simulink model "Fullorder_with_PID"  (R2015b)
settings: Solver=VariableStepAuto  StartTime=0.0  StopTime=10.0  RelTol=1e-3
undefined symbols (not defined in the file): J_pro, Kt, Kv, L, R
libraries: simulink x1
settings Model: Creator=Morten  LastModifiedBy=Morten

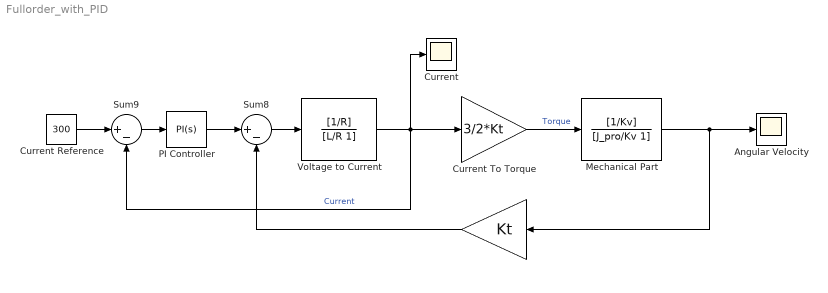
== system Fullorder_with_PID ==
  "                " : Gain  Gain=Kt
  Angular Velocity : Scope
  Current : Scope
  Current Reference : Constant  Value=300
  "Current To Torque " : Gain  Gain=3/2*Kt
  "Mechanical Part " : TransferFcn  Numerator=[1/Kv]  Denominator=[J_pro/Kv 1]
  "PI Controller " : simulink/Continuous/PID Controller  Controller=PI  TimeDomain=Continuous-time  SampleTime=-1  IntegratorMethod=Forward Euler  FilterMethod=Forward Euler  Form=Parallel  UseFilter=on  ControllerParametersSource=internal  P=0.0157  I=2.5637  D=0  N=100  InitialConditionSource=internal  InitialConditionForIntegrator=0  InitialConditionForFilter=0  ExternalReset=none  LimitOutput=off  UpperSaturationLimit=inf  LowerSaturationLimit=-inf  LinearizeAsGain=on  AntiWindupMode=none  Kb=1  TrackingMode=off  Kt=1  PParamMin=[]  PParamMax=[]  IParamMin=[]  IParamMax=[]  DParamMin=[]  DParamMax=[]  NParamMin=[]  NParamMax=[]  KbParamMin=[]  KbParamMax=[]  KtParamMin=[]  KtParamMax=[]  POutMin=[]  POutMax=[]  IOutMin=[]  IOutMax=[]  DOutMin=[]  DOutMax=[]  NOutMin=[]  NOutMax=[]  KbOutMin=[]  KbOutMax=[]  KtOutMin=[]  KtOutMax=[]  IntegratorOutMin=[]  IntegratorOutMax=[]  FilterOutMin=[]  FilterOutMax=[]  SumOutMin=[]  SumOutMax=[]  SumI1OutMin=[]  SumI1OutMax=[]  SumI2OutMin=[]  SumI2OutMax=[]  SumI3OutMin=[]  SumI3OutMax=[]  SumDOutMin=[]  SumDOutMax=[]  SaturationOutMin=[]  SaturationOutMax=[]  IntegratorContinuousStateAttributes=''  IntegratorStateMustResolveToSignalObject=off  IntegratorRTWStateStorageClass=Auto  FilterContinuousStateAttributes=''  FilterStateMustResolveToSignalObject=off  FilterRTWStateStorageClass=Auto  DifferentiatorICPrevScaledInput=0  DifferentiatorOutMin=[]  DifferentiatorOutMax=[]
  Sum8 : Sum  Inputs=|+-
  Sum9 : Sum  Inputs=|+-
  "Voltage to Current " : TransferFcn  Numerator=[1/R]  Denominator=[L/R 1]
  wires:
  "                "/1 -> Sum8/2
  Sum8/1 -> "Voltage to Current "/1
  "Mechanical Part "/1 -> Angular Velocity/1, "                "/1
  Current Reference/1 -> Sum9/1
  "Voltage to Current "/1 -> Current/1, "Current To Torque "/1, Sum9/2  "Current"
  "Current To Torque "/1 -> "Mechanical Part "/1  "Torque"
  "PI Controller "/1 -> Sum8/1
  Sum9/1 -> "PI Controller "/1
